simulink model "actividad1_2simulink"  (R2021a)
settings: Solver=ode1  StartTime=0.0  StopTime=3  FixedStep=0.001  RelTol=1e-3
settings Model: Creator=Agus  LastModifiedBy=Agus

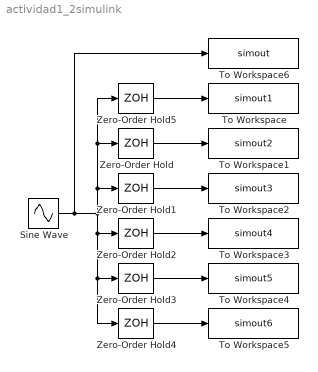
== system actividad1_2simulink ==
  Sine Wave : Sin  Frequency=2*pi  SampleTime=0
  To Workspace : ToWorkspace  VariableName=simout1  SampleTime=-1
  To Workspace1 : ToWorkspace  VariableName=simout2  SampleTime=-1
  To Workspace2 : ToWorkspace  VariableName=simout3  SampleTime=-1
  To Workspace3 : ToWorkspace  VariableName=simout4  SampleTime=-1
  To Workspace4 : ToWorkspace  VariableName=simout5  SampleTime=-1
  To Workspace5 : ToWorkspace  VariableName=simout6  SampleTime=-1
  To Workspace6 : ToWorkspace  VariableName=simout  SampleTime=-1
  Zero-Order Hold : ZeroOrderHold  SampleTime=0.5
  Zero-Order Hold1 : ZeroOrderHold  SampleTime=0.2
  Zero-Order Hold2 : ZeroOrderHold  SampleTime=0.1
  Zero-Order Hold3 : ZeroOrderHold  SampleTime=0.05
  Zero-Order Hold4 : ZeroOrderHold  SampleTime=0.01
  Zero-Order Hold5 : ZeroOrderHold  SampleTime=0.75
  wires:
  Sine Wave/1 -> To Workspace6/1, Zero-Order Hold5/1, Zero-Order Hold/1, Zero-Order Hold1/1, Zero-Order Hold4/1, Zero-Order Hold3/1, Zero-Order Hold2/1
  Zero-Order Hold5/1 -> To Workspace/1
  Zero-Order Hold/1 -> To Workspace1/1
  Zero-Order Hold1/1 -> To Workspace2/1
  Zero-Order Hold2/1 -> To Workspace3/1
  Zero-Order Hold3/1 -> To Workspace4/1
  Zero-Order Hold4/1 -> To Workspace5/1
